simulink model "imp"  (R2017a)
settings: Solver=ode45  StartTime=0.2  StopTime=6  MaxStep=.01  MinStep=.001  RelTol=1e-4  AbsTol=1e-4
values from neighbouring files (symbols this model uses):
  A = [-c(i)/M -k/M c(i)/M k/M ... (first row only)    [Quater_car.m]    (also in half_car.m = [-(cf(i)+cr(i))/M -(kf+kr)/M     cf(i)/M      kf/M     cr(i))
  B = [zeros(3,4)         , ... (first row only)    [Codefile.m]    (also in Quater_car.m = [0;0;kt/m;0]; half_car.m = [0 0 0;0 0 0;kt/mf 0 0;0 0 0;0 kt/mr 0;0 0 0;0 0 1/Iy;0 0 0])
undefined symbols (not defined in the file or in its folder): A1, C, E, K
settings Model: Creator=Gupta  LastModifiedBy=Gupta
settings SolverCC: InitialStep=.001

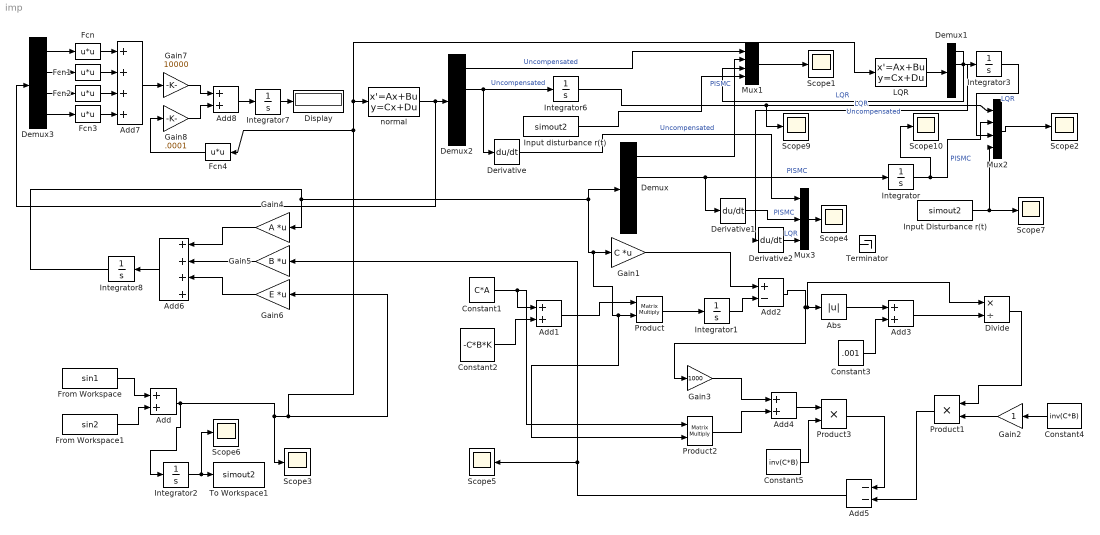
== system imp ==
  Abs : Abs
  Add{,1,3..4,8} (5 alike) : Sum
  Add2 : Sum  Inputs=+-
  Add5 : Sum  Inputs=--
  Add6 : Sum  Inputs=++++
  Add7 : Sum  Inputs=++++
  Constant1 : Constant  Value=C*A  VectorParams1D=off
  Constant2 : Constant  Value=-C*B*K  VectorParams1D=off
  Constant3 : Constant  Value=.001
  Constant4 : Constant  Value=inv(C*B)  VectorParams1D=off
  Constant5 : Constant  Value=inv(C*B)  VectorParams1D=off
  Demux{,1..3} (4 alike) : Demux
  Derivative : Derivative
  Derivative1 : Derivative
  Derivative2 : Derivative
  Display : Display
  Divide : Product  Inputs=*/
  Fcn{,1..4} (5 alike) : Fcn  Expr=u*u
  From Workspace : FromWorkspace  VariableName=sin1  SampleTime=0  Interpolate=off  OutputAfterFinalValue=Setting to zero
  From Workspace1 : FromWorkspace  VariableName=sin2  SampleTime=0  Interpolate=off  OutputAfterFinalValue=Setting to zero
  Gain1 : Gain  Gain=C  Multiplication=Matrix(K*u)
  Gain2 : Gain
  Gain3 : Gain  Gain=1000
  Gain4 : Gain  Gain=A  Multiplication=Matrix(K*u)
  Gain5 : Gain  Gain=B  Multiplication=Matrix(K*u)
  Gain6 : Gain  Gain=E  Multiplication=Matrix(K*u)
  Gain7 : Gain  Gain=10000
  Gain8 : Gain  Gain=.0001
  Input Disturbance r(t) : FromWorkspace  VariableName=simout2  Interpolate=off  OutputAfterFinalValue=Setting to zero
  Input disturbance r(t) : FromWorkspace  VariableName=simout2  Interpolate=off  OutputAfterFinalValue=Setting to zero
  Integrator{,1..3,6..8} (7 alike) : Integrator
  LQR : StateSpace  A=A1  B=[E]  C=eye(4)  D=zeros(4,1)  X0=0
  Mux1 : Mux
  Mux2 : Mux
  Mux3 : Mux  Inputs=3
  Product : Product  Multiplication=Matrix(*)
  Product1 : Product
  Product2 : Product  Multiplication=Matrix(*)
  Product3 : Product
  Scope{1..7,9..10} (9 alike) : Scope
  Terminator : Terminator
  To Workspace1 : ToWorkspace  VariableName=simout2  SaveFormat=Timeseries  SampleTime=-1
  normal : StateSpace  A=A  B=[E]  C=eye(4)  D=zeros(4,1)  X0=0
  wires:
  From Workspace/1 -> Add/1
  Demux/2 -> Derivative1/1, Integrator/1  "PISMC"
  Demux/1 -> Mux1/2  "PISMC"
  Integrator8/1 -> Demux/1, Product2/2, Product/2, Gain1/1, Gain4/1
  From Workspace1/1 -> Add/2
  Constant1/1 -> Product2/1, Add1/1
  Constant2/1 -> Add1/2
  Gain1/1 -> Add2/1
  Add2/1 -> Gain3/1, Divide/1, Abs/1
  Abs/1 -> Add3/1
  Add1/1 -> Product/1
  Constant3/1 -> Add3/2
  Add3/1 -> Divide/2
  Constant4/1 -> Gain2/1
  Gain2/1 -> Product1/2
  Divide/1 -> Product1/1
  Product2/1 -> Add4/2
  Add4/1 -> Product3/1
  Constant5/1 -> Product3/2
  Product3/1 -> Add5/1
  Product1/1 -> Add5/2
  Gain5/1 -> Add6/2
  Gain4/1 -> Add6/1
  Gain6/1 -> Add6/3
  Add6/1 -> Integrator8/1
  Add5/1 -> Scope5/1, Gain5/1
  Demux2/2 -> Integrator6/1, Derivative/1  "Uncompensated"
  Integrator6/1 -> Scope9/1, Mux2/1  "Uncompensated"
  normal/1 -> Demux2/1, Demux3/1
  Demux2/1 -> Mux1/1  "Uncompensated"
  Integrator/1 -> Scope10/1, Mux2/2  "PISMC"
  Mux1/1 -> Scope1/1
  Mux2/1 -> Scope2/1
  Demux3/1 -> Fcn/1
  Demux3/2 -> Fcn1/1
  Demux3/4 -> Fcn3/1
  Demux3/3 -> Fcn2/1
  Fcn/1 -> Add7/1
  Fcn1/1 -> Add7/2
  Fcn2/1 -> Add7/3
  Fcn3/1 -> Add7/4
  Add7/1 -> Gain7/1
  Gain7/1 -> Add8/1
  Gain8/1 -> Add8/2
  Add8/1 -> Integrator7/1
  Integrator7/1 -> Display/1
  Integrator2/1 -> Scope6/1, To Workspace1/1
  Input Disturbance r(t)/1 -> Mux2/4, Scope7/1
  Integrator1/1 -> Add2/2
  Product/1 -> Integrator1/1
  Gain3/1 -> Add4/1
  Input disturbance r(t)/1 -> Mux1/4
  LQR/1 -> Demux1/1
  Demux1/2 -> Derivative2/1, Integrator3/1  "LQR"
  Demux1/1 -> Mux1/3  "LQR"
  Integrator3/1 -> Mux2/3  "LQR"
  Mux3/1 -> Scope4/1
  Derivative/1 -> Mux3/1  "Uncompensated"
  Derivative1/1 -> Mux3/2  "PISMC"
  Derivative2/1 -> Mux3/3  "LQR"
  Add/1 -> Integrator2/1, Fcn4/1, normal/1, LQR/1, Gain6/1, Scope3/1
  Fcn4/1 -> Gain8/1
